simulink library "aerolib6dof"  (Simulink 5.0)
undefined symbols (not defined in the file or in its folder): e0_0, e1_0, e2_0, e3_0
libraries: aerolibtransform x8, aerolibutil x1, simulink3 x1
settings Model: ForwardingTableString=||__slOldName__||aerolib6dof/6DoF (Quaternion)||__slNewName__||aerolibprivatev1p5/6DoF (Quaternion)||__slOldName__||aerolib6dof/6DoF (Euler Angles)||__slNewName__||aerolibprivatev1p5/6DoF (Euler Angles)  Creator=sgage  LastModifiedBy=sgage  ExtModeAutoUpdateStatusClock=off  TargetHWChar=2  TargetHWWordLengths=8,16,32,32

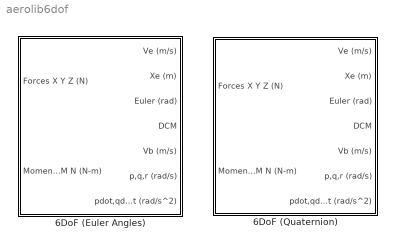
== system aerolib6dof ==
  6DoF (Euler Angles) : Subsystem  mask(6DoF (Euler Angles) EoM){xme_0=[0 0 0], Vm_0=[0 0 0], eul_0=[0 0 0], pm_0=[0 0 0], Mass=1.0, Inertia=eye(3)}
      mask prompts: xme_0 "Initial position in inertial axes [Xe,Ye,Ze] (m):"; Vm_0 "Initial velocity in body axes [U,v,w] (m/s):"; eul_0 "Initial Euler orientation [roll, pitch, yaw] (rad):"; pm_0 "Initial body rotation rates [p,q,r] (rad/s):"; Mass "Mass (kg):"; Inertia "Inertia matrix (kg.m^2):"
      mask help:
      | Integrate the six-degrees-of-freedom equations of motion using an Euler angle representation for the orientation of the body in space.
      |
      | Inputs are forces on the body in x-axis, y-axis, and z-axis; and moments on the body along x-axis, y-axis, and z-axis. Outputs are translational velocity in x-axis, y-axis, and z-axis in inertial coordinates; position in x-axis, y-axis, and z-axis in inertial coordinates; phi, theta, and psi; 3-by-3 direction cosine matrix; translational velocity in x-axis, y-axis, and z-axis in body coordinates; roll, pitch, and yaw rate; and roll, pitch, and yaw acceleration.
      mask Help: web(asbhelp('6dofeulerangles'));
      mask Display: disp('Euler\nAngles')
  6DoF (Quaternion) : Subsystem  mask(6DoF (Quaternion) EoM){xme_0=[0 0 0], Vm_0=[0 0 0], eul_0=[0 0 0], pm_0=[0 0 0], Mass=1.0, Inertia=eye(3), k_quat=1}
      mask prompts: xme_0 "Initial position in inertial axes [Xe,Ye,Ze] (m):"; Vm_0 "Initial velocity in body axes [U,v,w] (m/s):"; eul_0 "Initial Euler orientation [roll, pitch, yaw] (rad):"; pm_0 "Initial body rotation rates [p,q,r] (rad/s):"; Mass "Mass (kg):"; Inertia "Inertia matrix (kg.m^2):"; k_quat "Gain for quaternion normalization:"
      mask help:
      | Integrate the six-degrees-of-freedom equations of motion using a quaternion representation for the orientation of the body in space.
      |
      | Inputs are forces on the body in x-axis, y-axis, and z-axis; and moments on the body along x-axis, y-axis, and z-axis. Outputs are translational velocity in x-axis, y-axis, and z-axis in inertial coordinates; position in x-axis, y-axis, and z-axis in inertial coordinates; phi, theta, and psi; 3-by-3 direction cosine matrix; translational velocity in x-axis, y-axis, and z-axis in body coordinates; roll, pitch, and yaw rate; and roll, pitch, and yaw acceleration.
      mask Help: web(asbhelp('6dofquaternion'))
      mask Display: disp('Quaternions')

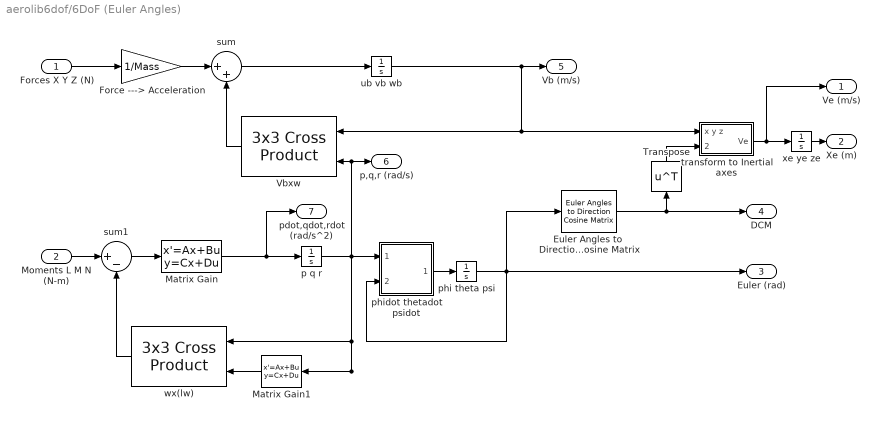
== system aerolib6dof/6DoF (Euler Angles) ==
  Forces X Y Z (N) : Inport  ShowAdditionalParam=on  DataType=double
  Moments L M N (N-m) : Inport  Port=2  ShowAdditionalParam=on  DataType=double
  Euler Angles to  Direction Cosine Matrix : aerolibtransform/Euler Angles to  Direction Cosine Matrix
  Force ---> Acceleration : Gain  Gain=1/Mass  SaturateOnIntegerOverflow=on
  Matrix Gain : StateSpace  A=[]  B=[]  C=[]  D=K  mask(Matrix Gain){@1=inv(Inertia)}
      mask prompts: @1 "Gain matrix:"
      mask help: Matrix Gain.
      mask init:
      | K = @1;
      mask Help: web(asbhelp);
      mask Display: disp('Inertia^(-1)')
  Matrix Gain1 : StateSpace  Orientation=left  A=[]  B=[]  C=[]  D=K  mask(Matrix Gain){@1=Inertia}
      mask prompts: @1 "Gain matrix:"
      mask help: Matrix Gain.
      mask init:
      | K = @1;
      mask Help: Multiplies input vector by entered matrix to produce output vector (y=Au).
      mask Display: disp('Inertia')
  Transpose : Math  Orientation=up  Operator=transpose
  Vbxw : aerolibtransform/3x3 Cross Product  Orientation=left
  p q r : Integrator  InitialCondition=pm_0
  phi theta psi : Integrator  InitialCondition=eul_0
  phidot thetadot psidot : Subsystem
  sum : Sum  Inputs=|++  SaturateOnIntegerOverflow=on  InputSameDT=on
  sum1 : Sum  Inputs=|+-  SaturateOnIntegerOverflow=on  InputSameDT=on
  "transform to Inertial axes " : Subsystem
      mask Type: Vector Transformation
      mask Display: disp('L_EB')
  ub vb wb : Integrator  InitialCondition=Vm_0
  wx(lw) : aerolibtransform/3x3 Cross Product  Orientation=left
  xe ye ze : Integrator  InitialCondition=xme_0
  Ve (m/s) : Outport
  Xe (m) : Outport  Port=2
  Euler (rad) : Outport  Port=3
  DCM : Outport  Port=4
  Vb (m/s) : Outport  Port=5
  p,q,r (rad/s) : Outport  Port=6
  pdot,qdot,rdot (rad/s^2) : Outport  Port=7
  wires:
  phidot thetadot psidot/1(phidot thetadot psi) -> phi theta psi/1
  phi theta psi/1 -> Euler (rad)/1, Euler Angles to  Direction Cosine Matrix/1, phidot thetadot psidot/2(phi theta psi)
  ub vb wb/1 -> Vb (m/s)/1, Vbxw/1, "transform to Inertial axes "/1(x y z)
  sum/1 -> ub vb wb/1
  xe ye ze/1 -> Xe (m)/1
  "transform to Inertial axes "/1(Ve) -> Ve (m/s)/1, xe ye ze/1
  p q r/1 -> p,q,r (rad/s)/1, Vbxw/2, wx(lw)/1, Matrix Gain1/1, phidot thetadot psidot/1(p q r)
  sum1/1 -> Matrix Gain/1
  Moments L M N (N-m)/1 -> sum1/1
  Matrix Gain1/1 -> wx(lw)/2
  wx(lw)/1 -> sum1/2
  Matrix Gain/1 -> pdot,qdot,rdot (rad/s^2)/1, p q r/1
  Forces X Y Z (N)/1 -> Force ---> Acceleration/1
  Vbxw/1 -> sum/2
  Force ---> Acceleration/1 -> sum/1
  Euler Angles to  Direction Cosine Matrix/1 -> DCM/1, Transpose/1
  Transpose/1 -> "transform to Inertial axes "/2(transform coefficients)

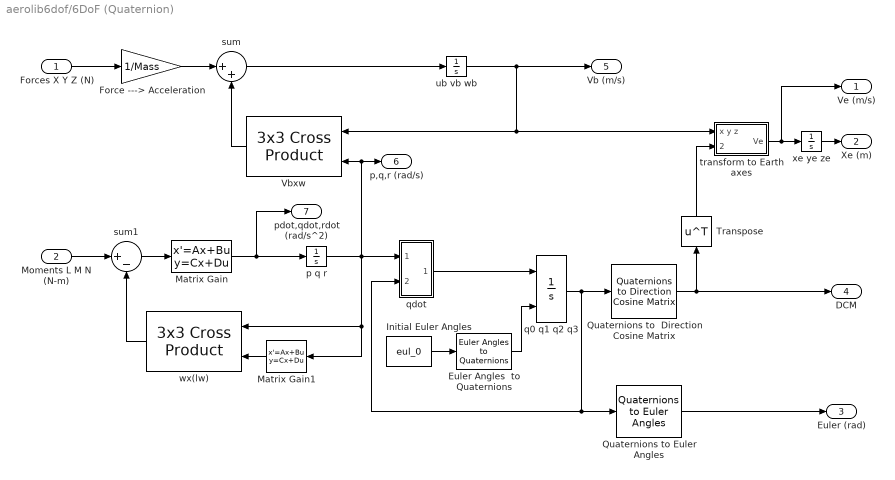
== system aerolib6dof/6DoF (Quaternion) ==
  Forces X Y Z (N) : Inport  ShowAdditionalParam=on  DataType=double
  Moments L M N (N-m) : Inport  Port=2  ShowAdditionalParam=on  DataType=double
  Euler Angles  to Quaternions : aerolibtransform/Euler Angles to Quaternions
  Force ---> Acceleration : Gain  Gain=1/Mass  SaturateOnIntegerOverflow=on
  Initial Euler Angles : Constant  Value=eul_0
  Matrix Gain : StateSpace  A=[]  B=[]  C=[]  D=K  mask(Matrix Gain){@1=inv(Inertia)}
      mask prompts: @1 "Gain matrix:"
      mask help: Matrix Gain.
      mask init:
      | K = @1;
      mask Help: Multiplies input vector by entered matrix to produce output vector (y=Au).
      mask Display: disp('Inertia^(-1)')
  Matrix Gain1 : StateSpace  Orientation=left  A=[]  B=[]  C=[]  D=K  mask(Matrix Gain){@1=Inertia}
      mask prompts: @1 "Gain matrix:"
      mask help: Matrix Gain.
      mask init:
      | K = @1;
      mask Help: Multiplies input vector by entered matrix to produce output vector (y=Au).
      mask Display: disp('Inertia')
  Quaternions to  Direction Cosine Matrix : aerolibtransform/Quaternions to  Direction Cosine Matrix
  Quaternions to Euler Angles : aerolibtransform/Quaternions to Euler Angles
  Transpose : Math  Orientation=up  Operator=transpose
  Vbxw : aerolibtransform/3x3 Cross Product  Orientation=left
  p q r : Integrator  InitialCondition=pm_0
  q0 q1 q2 q3 : Integrator  InitialConditionSource=external  InitialCondition=[e0_0 e1_0 e2_0 e3_0]
  qdot : Subsystem
  sum : Sum  Inputs=|++  SaturateOnIntegerOverflow=on  InputSameDT=on
  sum1 : Sum  Inputs=|+-  SaturateOnIntegerOverflow=on  InputSameDT=on
  "transform to Earth axes " : Subsystem
      mask Type: Vector Transformation
      mask Display: disp('L_EB')
  ub vb wb : Integrator  InitialCondition=Vm_0
  wx(lw) : aerolibtransform/3x3 Cross Product  Orientation=left
  xe ye ze : Integrator  InitialCondition=xme_0
  Ve (m/s) : Outport
  Xe (m) : Outport  Port=2
  Euler (rad) : Outport  Port=3
  DCM : Outport  Port=4
  Vb (m/s) : Outport  Port=5
  p,q,r (rad/s) : Outport  Port=6
  pdot,qdot,rdot (rad/s^2) : Outport  Port=7
  wires:
  Quaternions to  Direction Cosine Matrix/1 -> DCM/1, Transpose/1
  Quaternions to Euler Angles/1 -> Euler (rad)/1
  p q r/1 -> qdot/1(p q r), Vbxw/2, p,q,r (rad/s)/1, wx(lw)/1, Matrix Gain1/1
  sum1/1 -> Matrix Gain/1
  Moments L M N (N-m)/1 -> sum1/1
  Matrix Gain1/1 -> wx(lw)/2
  wx(lw)/1 -> sum1/2
  qdot/1(qdot) -> q0 q1 q2 q3/1
  q0 q1 q2 q3/1 -> qdot/2(q0 q1 q2 q3), Quaternions to Euler Angles/1, Quaternions to  Direction Cosine Matrix/1
  Matrix Gain/1 -> p q r/1, pdot,qdot,rdot (rad/s^2)/1
  ub vb wb/1 -> Vbxw/1, "transform to Earth axes "/1(x y z), Vb (m/s)/1
  Forces X Y Z (N)/1 -> Force ---> Acceleration/1
  Vbxw/1 -> sum/2
  sum/1 -> ub vb wb/1
  Force ---> Acceleration/1 -> sum/1
  xe ye ze/1 -> Xe (m)/1
  "transform to Earth axes "/1(Ve) -> xe ye ze/1, Ve (m/s)/1
  Transpose/1 -> "transform to Earth axes "/2(transform coefficients)
  Euler Angles  to Quaternions/1 -> q0 q1 q2 q3/2
  Initial Euler Angles/1 -> Euler Angles  to Quaternions/1

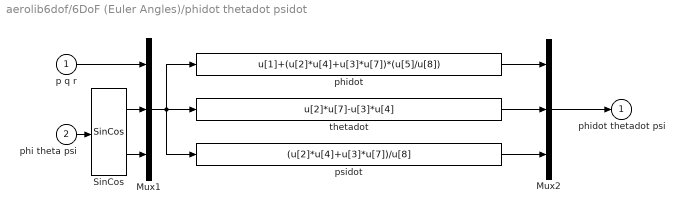
== system aerolib6dof/6DoF (Euler Angles)/phidot thetadot psidot ==
  p q r : Inport
  phi theta psi : Inport  Port=2
  Mux1 : Mux  Inputs=[3 3 3]
  Mux2 : Mux  Inputs=3
  SinCos : aerolibutil/SinCos
  phidot : Fcn  Expr=u[1]+(u[2]*u[4]+u[3]*u[7])*(u[5]/u[8])
  psidot : Fcn  Expr=(u[2]*u[4]+u[3]*u[7])/u[8]
  thetadot : Fcn  Expr=u[2]*u[7]-u[3]*u[4]
  phidot thetadot psi : Outport  InitialOutput=0
  wires:
  Mux1/1 -> psidot/1, phidot/1, thetadot/1
  p q r/1 -> Mux1/1
  phi theta psi/1 -> SinCos/1
  psidot/1 -> Mux2/3
  thetadot/1 -> Mux2/2
  phidot/1 -> Mux2/1
  Mux2/1 -> phidot thetadot psi/1
  SinCos/1 -> Mux1/2
  SinCos/2 -> Mux1/3

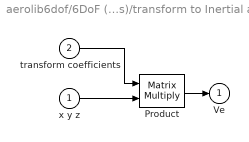
== system aerolib6dof/6DoF (Euler Angles)/transform to Inertial axes  ==
  x y z : Inport
  transform coefficients : Inport  Port=2
  Product : Product  Multiplication=Matrix(*)  SaturateOnIntegerOverflow=on  InputSameDT=on
  Ve : Outport  InitialOutput=0
  wires:
  x y z/1 -> Product/2
  transform coefficients/1 -> Product/1
  Product/1 -> Ve/1

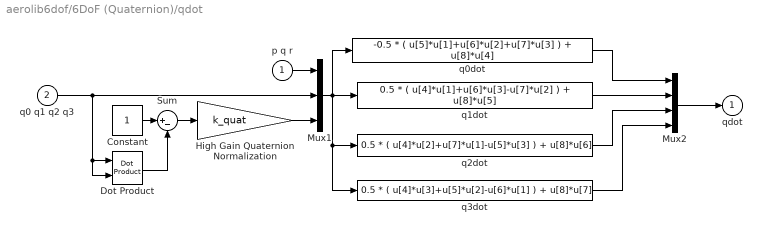
== system aerolib6dof/6DoF (Quaternion)/qdot ==
  p q r : Inport
  q0 q1 q2 q3 : Inport  Port=2
  Constant : Constant
  Dot Product : simulink3/Math/Dot Product
  High Gain Quaternion Normalization : Gain  Gain=k_quat  SaturateOnIntegerOverflow=on
  Mux1 : Mux  Inputs=[3 4 1]
  Mux2 : Mux
  Sum : Sum  Inputs=|+-  SaturateOnIntegerOverflow=on  InputSameDT=on
  q0dot : Fcn  Expr=-0.5 * ( u[5]*u[1]+u[6]*u[2]+u[7]*u[3] ) + u[8]*u[4]
  q1dot : Fcn  Expr=0.5 * ( u[4]*u[1]+u[6]*u[3]-u[7]*u[2] ) + u[8]*u[5]
  q2dot : Fcn  Expr=0.5 * ( u[4]*u[2]+u[7]*u[1]-u[5]*u[3] ) + u[8]*u[6]
  q3dot : Fcn  Expr=0.5 * ( u[4]*u[3]+u[5]*u[2]-u[6]*u[1] ) + u[8]*u[7]
  qdot : Outport  InitialOutput=0
  wires:
  p q r/1 -> Mux1/1
  Dot Product/1 -> Sum/2
  High Gain Quaternion Normalization/1 -> Mux1/3
  Sum/1 -> High Gain Quaternion Normalization/1
  Constant/1 -> Sum/1
  Mux2/1 -> qdot/1
  q0dot/1 -> Mux2/1
  q1dot/1 -> Mux2/2
  q2dot/1 -> Mux2/3
  Mux1/1 -> q2dot/1, q3dot/1, q0dot/1, q1dot/1
  q3dot/1 -> Mux2/4
  q0 q1 q2 q3/1 -> Dot Product/1, Dot Product/2, Mux1/2

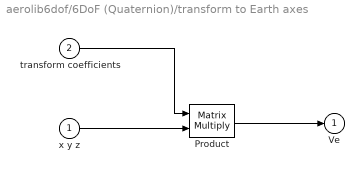
== system aerolib6dof/6DoF (Quaternion)/transform to Earth axes  ==
  x y z : Inport
  transform coefficients : Inport  Port=2
  Product : Product  Multiplication=Matrix(*)  SaturateOnIntegerOverflow=on  InputSameDT=on
  Ve : Outport  InitialOutput=0
  wires:
  Product/1 -> Ve/1
  transform coefficients/1 -> Product/1
  x y z/1 -> Product/2
